simulink model "Leg"  (R2022a)
settings: Solver=VariableStepAuto  StartTime=0.0  StopTime=StopTime  FixedStep=0.001  MinStep=0.005  RelTol=1e-3
values from neighbouring files (symbols this model uses):
  l1 = 0.24    [thet_B.m]    (also in thet_S.m)
  l2 = 1.5    [thet_B.m]    (also in thet_S.m)
  l3 = 1.2    [thet_B.m]    (also in thet_S.m)
  l4 = 0.56    [thet_B.m]    (also in thet_S.m)
  s = size(theta_shag,1)    [Thetas.m]    (also in thet_B.m = size(sim_B.footPos,2); thet_P.m = size(sim_P.footPos,2); thet_S.m = size(simStates.footPos,2))
undefined symbols (not defined in the file or in its folder): L1, L2, L3, L4, m1, m2, m3, m4, mass_1, mass_2, mass_3, mass_4, X, Y, Z
libraries: nesl_utility x17, sm_lib x16
settings Model: Creator=boris_1863  LastModifiedBy=180
settings SolverCC: AlgebraicLoopSolver=TrustRegion
settings DataIOCC: MaxDataPoints=10000  ReturnWorkspaceOutputs=off  OutputTimes=0:0.01:StopTime
settings DebuggingCC: UnconnectedInputMsg=warning  UnconnectedOutputMsg=warning  UnconnectedLineMsg=warning  SFMachineParentedDataDiag=warning
settings RTWCC: DLArmComputeVersion=19.05
settings DiagnosticsConfigSet: SimMechanicsInvalidVisualProperty=none  SimMechanicsCrossSectionNullEdge=none  SimMechanicsUnconnectedFramePorts=none  SimMechanicsUnconnectedGeometryPorts=none  SimMechanicsRedundantBlock=none  SimMechanicsConflictingReferenceFrames=none  SimMechanicsRigidlyBoundBlock=none  SimMechanicsUnsatisfiedHighPriorityTargets=none  SimMechanicsJointTargetOverSpecification=none
settings ExplorerConfigSet: InternalSimMechanicsExplorerSettings="<ExplorerConfiguration><canonicalview>default</canonicalview><AnimationSetting><BasePlaybackSpeed>1.0</BasePlaybackSpeed><PlaybackSpeedFactor>4.0</PlaybackSpeedFactor></AnimationSetting><TilePanel><TileInfo><Tiles Columns=\"1\" Count=\"1\" Rows=\"1\"><Column Weight=\"1\"/><Row Weight=\"1\"/><Tile Height=\"1\" Width=\"1\" X=\"0\" Y=\"0\"/></Tiles></TileInfo><SceneInfo><SceneViewer><BGColor><R>1</R><G>1</G><B>1</B></BGColor><Camera><DoPerspective>off</DoPerspective><Position><X>0.0567000060216437882</X><Y>-1</Y><Z>0.046455009033208941</Z></Position><Center><X>0.0567000060216437882</X><Y>0</Y><Z>0.046455009033208941</Z></Center><Up><X>0</X><Y>-0</Y><Z>1</Z></Up><ViewLimDist>1</ViewLimDist><YLim>0.243616639058569923</YLim><XLim>0.23167689803025171</XLim></Camera></SceneViewer></SceneInfo></TilePanel><MechEditorPanel><Cameras/><GfxPanelCameraMap/><VideoCreator><PlaybackSpeedRatio>0.5</PlaybackSpeedRatio><FrameRate>60</FrameRate><VideoFormat>MPEG-4</VideoFormat><FrameSize>auto</FrameSize></VideoCreator></MechEditorPanel></ExplorerConfiguration>"

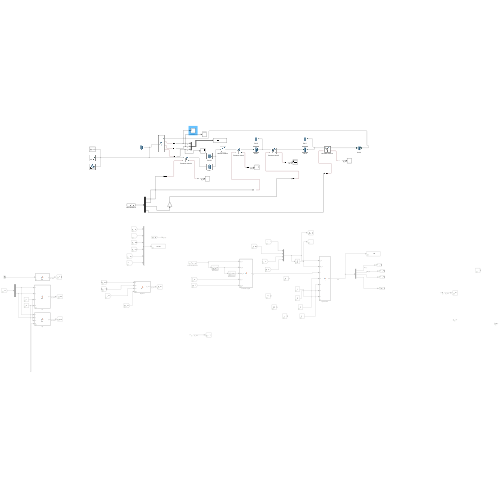
[thumbnail: Simulink's stored preview of the top-level diagram]
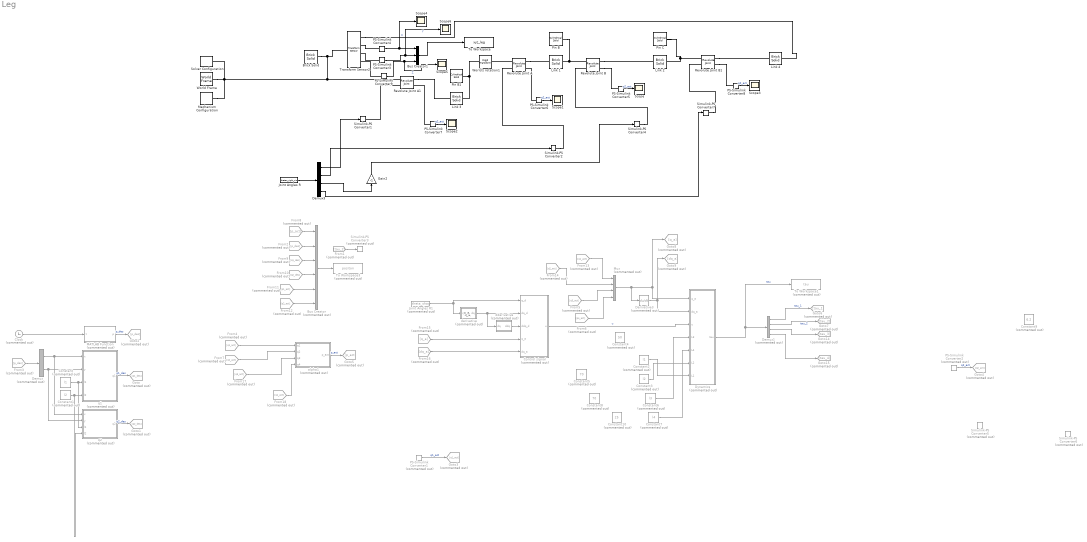
== system Leg ==
  note: q_a,
  note: q_a,
  Brick Solid : sm_lib/Body Elements/Brick Solid  GraphicAmbientColor=[0.15 0.15 0.15 1.0]  BasedOnType=Density  BrickDimensions=[0.12 0.12 0.12]  BrickDimensionUnits=m  CenterOfMass=[0 0 0]  CenterOfMassUnits=m  GraphicDiffuseColor=[0.2 0.2 0.2]  Density=1000  DensityUnits=kg/m^3  DoExposeReferenceFrame=on  GraphicEmissiveColor=[0.0 0.0 0.0 1.0]  ExportEntireGeometry=off  SerializedFrames=<Frames/>  MarkerShape=Sphere  MarkerSize=10  GraphicType=FromGeometry  InertiaType=CalculateFromGeometry  Mass=1  MassUnits=kg  MomentsOfInertia=[1 1 1]  MomentsOfInertiaUnits=kg*m^2  GraphicOpacity=1.0  ProductsOfInertia=[0 0 0]  ProductsOfInertiaUnits=kg*m^2  GraphicShininess=75  GraphicSpecularColor=[0.5 0.5 0.5 1.0]  GraphicVisPropType=SimpleVisualProperties
  Bus Creator : BusCreator  Commented=on  Inputs=6
  Bus Creator1 : BusCreator  Inputs=3
  Clock : Clock  Commented=on
  Constant : Constant  Commented=on  Value=l1
  Constant1 : Constant  Commented=on  Value=l2
  Constant10 : Constant  Commented=on  Value=25
  Constant2 : Constant  Commented=on  Value=l1
  Constant3 : Constant  Commented=on  Value=l2
  Constant4 : Constant  Commented=on  Value=50
  Constant5 : Constant  Commented=on  Value=70
  Constant6 : Constant  Commented=on  Value=l3
  Constant7 : Constant  Commented=on  Value=l4
  Constant8 : Constant  Commented=on  Value=70
  Constant9 : Constant  Commented=on  Value=6.2
  Control signal : MATLAB Function  Commented=on  TreatAsAtomicUnit=on
  Demux : Demux  Commented=on  Outputs=2
  Demux1 : Demux  Commented=on
  Demux3 : Demux
  Derivative3 : Derivative  Commented=on
  Dynamics : MATLAB Function  Commented=on  TreatAsAtomicUnit=on
  From1 : From  Commented=on  GotoTag=tau_2
  From10 : From  Commented=on  GotoTag=q2_des
  From11 : From  Commented=on  GotoTag=q1_act
  From12 : From  Commented=on  GotoTag=q2_act
  From13 : From  Commented=on  GotoTag=q1_act
  From14 : From  Commented=on  GotoTag=q2_act
  From15 : From  Commented=on  GotoTag=q_a
  From16 : From  Commented=on  GotoTag=dq_a
  From17 : From  Commented=on  GotoTag=q3_act
  From18 : From  Commented=on  GotoTag=q4_act
  From2 : From  Commented=on  GotoTag=p_des
  From3 : From  Commented=on  GotoTag=p_des
  From4 : From  Commented=on  GotoTag=q1_act
  From5 : From  Commented=on  GotoTag=q3_act
  From6 : From  Commented=on  GotoTag=q4_act
  From7 : From  Commented=on  GotoTag=q2_act
  From8 : From  Commented=on  GotoTag=p_act
  From9 : From  Commented=on  GotoTag=q1_des
  Gain2 : Gain  Gain=-1
  Goto : Goto  Commented=on  GotoTag=q1_des
  Goto1 : Goto  Commented=on  GotoTag=q2_des
  Goto14 : Goto  Commented=on  GotoTag=tau_3
  Goto15 : Goto  Commented=on  GotoTag=tau_4
  Goto2 : Goto  Commented=on  GotoTag=p_des
  Goto3 : Goto  Commented=on  GotoTag=q1_act
  Goto4 : Goto  Commented=on  GotoTag=q2_act
  Goto5 : Goto  Commented=on  GotoTag=p_act
  Goto6 : Goto  Commented=on  GotoTag=tau_1
  Goto7 : Goto  Commented=on  GotoTag=tau_2
  Goto8 : Goto  Commented=on  GotoTag=q_a
  Goto9 : Goto  Commented=on  GotoTag=dq_a
  Joint Angles R : FromWorkspace  VariableName=thetas_right_niz  OutputAfterFinalValue=Holding final value
  Joint Angles R1 : FromWorkspace  Commented=on  VariableName=theta_shag  OutputAfterFinalValue=Holding final value
  Link 1 : sm_lib/Body Elements/Brick Solid  GraphicAmbientColor=[0.15 0.15 0.15 1.0]  BasedOnType=Mass  BrickDimensions=BC  BrickDimensionUnits=m  CenterOfMass=[0 0 0]  CenterOfMassUnits=m  GraphicDiffuseColor=[0.6 0.6 1.0]  Density=1000  DensityUnits=kg/m^3  DoExposeReferenceFrame=off  GraphicEmissiveColor=[0.0 0.0 0.0 1.0]  ExportEntireGeometry=off  SerializedFrames=<Frames><Frame><Id>Frame1</Id><Value><Name>F1</Name><Origin><Source>GeometricFeature</Source><FeatureName>-x surface</FeatureName></Origin><PrimaryAxis><DefinedDirection>+Z</DefinedDirection><Source>ReferenceFrame</Source><SourceDirection>+Z</SourceDirection><FeatureName></FeatureName></PrimaryAxis><SecondaryAxis><DefinedDirection>+X</DefinedDirection><Source>ReferenceFrame</Source><SourceDirection>+X</SourceDirection><FeatureName></FeatureName></SecondaryAxis></Value></Frame><Frame><Id>Frame2</Id><Value><Name>F2</Name><Origin><Source>GeometricFeature</Source><FeatureName>+x surface</FeatureName></Origin><PrimaryAxis><DefinedDirection>+Z</DefinedDirection><Source>ReferenceFrame</Source><SourceDirection>+Z</SourceDirection><FeatureName></FeatureName></PrimaryAxis><SecondaryAxis><DefinedDirection>+X</DefinedDirection><Source>ReferenceFrame</Source><SourceDirection>+X</SourceDirection><FeatureName></FeatureName></SecondaryAxis></Value></Frame></Frames>  MarkerShape=Sphere  MarkerSize=10  GraphicType=FromGeometry  InertiaType=PointMass  Mass=mass_2  MassUnits=kg  MomentsOfInertia=[1 1 1]  MomentsOfInertiaUnits=kg*m^2  GraphicOpacity=1.0  ProductsOfInertia=[0 0 0]  ProductsOfInertiaUnits=kg*m^2  GraphicShininess=75  GraphicSpecularColor=[0.5 0.5 0.5 1.0]  GraphicVisPropType=SimpleVisualProperties
  Link 2 : sm_lib/Body Elements/Brick Solid  GraphicAmbientColor=[0.15 0.15 0.15 1.0]  BasedOnType=Mass  BrickDimensions=CD  BrickDimensionUnits=m  CenterOfMass=[0 0 0]  CenterOfMassUnits=m  GraphicDiffuseColor=[0.2 0.2 1.0]  Density=1000  DensityUnits=kg/m^3  DoExposeReferenceFrame=off  GraphicEmissiveColor=[0.0 0.0 0.0 1.0]  ExportEntireGeometry=off  SerializedFrames=<Frames><Frame><Id>Frame1</Id><Value><Name>F1</Name><Origin><Source>GeometricFeature</Source><FeatureName>-x surface</FeatureName></Origin><PrimaryAxis><DefinedDirection>+Z</DefinedDirection><Source>ReferenceFrame</Source><SourceDirection>+Z</SourceDirection><FeatureName></FeatureName></PrimaryAxis><SecondaryAxis><DefinedDirection>+X</DefinedDirection><Source>ReferenceFrame</Source><SourceDirection>+X</SourceDirection><FeatureName></FeatureName></SecondaryAxis></Value></Frame><Frame><Id>Frame2</Id><Value><Name>F2</Name><Origin><Source>GeometricFeature</Source><FeatureName>+x surface</FeatureName></Origin><PrimaryAxis><DefinedDirection>+Z</DefinedDirection><Source>ReferenceFrame</Source><SourceDirection>+Z</SourceDirection><FeatureName></FeatureName></PrimaryAxis><SecondaryAxis><DefinedDirection>+X</DefinedDirection><Source>ReferenceFrame</Source><SourceDirection>+X</SourceDirection><FeatureName></FeatureName></SecondaryAxis></Value></Frame></Frames>  MarkerShape=Sphere  MarkerSize=10  GraphicType=FromGeometry  InertiaType=PointMass  Mass=mass_3  MassUnits=kg  MomentsOfInertia=[1 1 1]  MomentsOfInertiaUnits=kg*m^2  GraphicOpacity=1.0  ProductsOfInertia=[0 0 0]  ProductsOfInertiaUnits=kg*m^2  GraphicShininess=75  GraphicSpecularColor=[0.5 0.5 0.5 1.0]  GraphicVisPropType=SimpleVisualProperties
  Link 3 : sm_lib/Body Elements/Brick Solid  GraphicAmbientColor=[0.15 0.15 0.15 1.0]  BasedOnType=Mass  BrickDimensions=AB  BrickDimensionUnits=m  CenterOfMass=[0 0 0]  CenterOfMassUnits=m  GraphicDiffuseColor=[0.6 0.6 1.0]  Density=1000  DensityUnits=kg/m^3  DoExposeReferenceFrame=off  GraphicEmissiveColor=[0.0 0.0 0.0 1.0]  ExportEntireGeometry=off  SerializedFrames=<Frames><Frame><Id>Frame1</Id><Value><Name>F1</Name><Origin><Source>GeometricFeature</Source><FeatureName>-x surface</FeatureName></Origin><PrimaryAxis><DefinedDirection>+Z</DefinedDirection><Source>ReferenceFrame</Source><SourceDirection>+Z</SourceDirection><FeatureName></FeatureName></PrimaryAxis><SecondaryAxis><DefinedDirection>+X</DefinedDirection><Source>ReferenceFrame</Source><SourceDirection>+X</SourceDirection><FeatureName></FeatureName></SecondaryAxis></Value></Frame><Frame><Id>Frame2</Id><Value><Name>F2</Name><Origin><Source>GeometricFeature</Source><FeatureName>+x surface</FeatureName></Origin><PrimaryAxis><DefinedDirection>+Z</DefinedDirection><Source>ReferenceFrame</Source><SourceDirection>+Z</SourceDirection><FeatureName></FeatureName></PrimaryAxis><SecondaryAxis><DefinedDirection>+X</DefinedDirection><Source>ReferenceFrame</Source><SourceDirection>+X</SourceDirection><FeatureName></FeatureName></SecondaryAxis></Value></Frame></Frames>  MarkerShape=Sphere  MarkerSize=10  GraphicType=FromGeometry  InertiaType=PointMass  Mass=mass_1  MassUnits=kg  MomentsOfInertia=[1 1 1]  MomentsOfInertiaUnits=kg*m^2  GraphicOpacity=1.0  ProductsOfInertia=[0 0 0]  ProductsOfInertiaUnits=kg*m^2  GraphicShininess=75  GraphicSpecularColor=[0.5 0.5 0.5 1.0]  GraphicVisPropType=SimpleVisualProperties
  Link 4 : sm_lib/Body Elements/Brick Solid  GraphicAmbientColor=[0.15 0.15 0.15 1.0]  BasedOnType=Mass  BrickDimensions=DE  BrickDimensionUnits=m  CenterOfMass=[0 0 0]  CenterOfMassUnits=m  GraphicDiffuseColor=[0.2 0.2 1.0]  Density=1000  DensityUnits=kg/m^3  DoExposeReferenceFrame=off  GraphicEmissiveColor=[0.0 0.0 0.0 1.0]  ExportEntireGeometry=off  SerializedFrames=<Frames><Frame><Id>Frame1</Id><Value><Name>F1</Name><Origin><Source>GeometricFeature</Source><FeatureName>-x surface</FeatureName></Origin><PrimaryAxis><DefinedDirection>+Z</DefinedDirection><Source>ReferenceFrame</Source><SourceDirection>+Z</SourceDirection><FeatureName></FeatureName></PrimaryAxis><SecondaryAxis><DefinedDirection>+X</DefinedDirection><Source>ReferenceFrame</Source><SourceDirection>+X</SourceDirection><FeatureName></FeatureName></SecondaryAxis></Value></Frame><Frame><Id>Frame2</Id><Value><Name>F2</Name><Origin><Source>GeometricFeature</Source><FeatureName>+x surface</FeatureName></Origin><PrimaryAxis><DefinedDirection>+Z</DefinedDirection><Source>ReferenceFrame</Source><SourceDirection>+Z</SourceDirection><FeatureName></FeatureName></PrimaryAxis><SecondaryAxis><DefinedDirection>+X</DefinedDirection><Source>ReferenceFrame</Source><SourceDirection>+X</SourceDirection><FeatureName></FeatureName></SecondaryAxis></Value></Frame></Frames>  MarkerShape=Sphere  MarkerSize=10  GraphicType=FromGeometry  InertiaType=PointMass  Mass=mass_4  MassUnits=kg  MomentsOfInertia=[1 1 1]  MomentsOfInertiaUnits=kg*m^2  GraphicOpacity=1.0  ProductsOfInertia=[0 0 0]  ProductsOfInertiaUnits=kg*m^2  GraphicShininess=75  GraphicSpecularColor=[0.5 0.5 0.5 1.0]  GraphicVisPropType=SimpleVisualProperties
  MATLAB Function : MATLAB Function  Commented=on  TreatAsAtomicUnit=on
  Mechanism Configuration : sm_lib/Utilities/Mechanism Configuration  UniformGravity=Constant  GravityVector=[0 0 -9.80665]  GravityUnits=m/s^2  LinearizationDelta=0.001  JointModeTransitionNonlinearIterations=2
  Mux : Mux  Commented=on
  PS-Simulink Converter1 : nesl_utility/PS-Simulink Converter  Commented=on  PhysicalDomain=network_engine_domain  SubClassName=ps_output  LeftPortType=input  RightPortType=output  PseudoPeriodic=off  Frequencies=[]  VectorFormat=1-D array  Unit=rad  AffineConversion=off
      settings: SourceProductBaseCode=SS,PW,VE
  PS-Simulink Converter2 : nesl_utility/PS-Simulink Converter  Commented=on  PhysicalDomain=network_engine_domain  SubClassName=ps_output  LeftPortType=input  RightPortType=output  PseudoPeriodic=off  Frequencies=[]  VectorFormat=1-D array  Unit=rad  AffineConversion=off
      settings: SourceProductBaseCode=SS,PW,VE
  PS-Simulink Converter3 : nesl_utility/PS-Simulink Converter  PhysicalDomain=network_engine_domain  SubClassName=ps_output  LeftPortType=input  RightPortType=output  PseudoPeriodic=off  Frequencies=[]  VectorFormat=1-D array  Unit=m  AffineConversion=off
      settings: SourceProductBaseCode=SS,PW,VE
  PS-Simulink Converter4 : nesl_utility/PS-Simulink Converter  PhysicalDomain=network_engine_domain  SubClassName=ps_output  LeftPortType=input  RightPortType=output  PseudoPeriodic=off  Frequencies=[]  VectorFormat=1-D array  Unit=m  AffineConversion=off
      settings: SourceProductBaseCode=SS,PW,VE
  PS-Simulink Converter{5..8} (4 alike) : nesl_utility/PS-Simulink Converter  PhysicalDomain=network_engine_domain  SubClassName=ps_output  LeftPortType=input  RightPortType=output  PseudoPeriodic=off  Frequencies=[]  VectorFormat=1-D array  Unit=rad  AffineConversion=off
      settings: SourceProductBaseCode=SS,PW,VE
  PS-Simulink Converter9 : nesl_utility/PS-Simulink Converter  PhysicalDomain=network_engine_domain  SubClassName=ps_output  LeftPortType=input  RightPortType=output  PseudoPeriodic=off  Frequencies=[]  VectorFormat=1-D array  Unit=m  AffineConversion=off
      settings: SourceProductBaseCode=SS,PW,VE
  Pin B : sm_lib/Body Elements/Cylindrical Solid  GraphicAmbientColor=[0.15 0.15 0.15 1.0]  BasedOnType=Density  CenterOfMass=[0 0 0]  CenterOfMassUnits=m  GraphicDiffuseColor=[0.6 0.6 1.0]  CylinderLength=0.11  CylinderLengthUnits=m  CylinderRadius=0.09/2  CylinderRadiusUnits=m  Density=0  DensityUnits=kg/m^3  DoExposeReferenceFrame=on  GraphicEmissiveColor=[0.0 0.0 0.0 1.0]  ExportEntireGeometry=off  SerializedFrames=<Frames/>  MarkerShape=Sphere  MarkerSize=10  GraphicType=FromGeometry  InertiaType=CalculateFromGeometry  Mass=1  MassUnits=kg  MomentsOfInertia=[1 1 1]  MomentsOfInertiaUnits=kg*m^2  GraphicOpacity=1.0  ProductsOfInertia=[0 0 0]  ProductsOfInertiaUnits=kg*m^2  GraphicShininess=75  GraphicSpecularColor=[0.5 0.5 0.5 1.0]  GraphicVisPropType=SimpleVisualProperties
  Pin B1 : sm_lib/Body Elements/Cylindrical Solid  GraphicAmbientColor=[0.15 0.15 0.15 1.0]  BasedOnType=Density  CenterOfMass=[0 0 0]  CenterOfMassUnits=m  GraphicDiffuseColor=[0.6 0.6 1.0]  CylinderLength=0.11  CylinderLengthUnits=m  CylinderRadius=0.09/2  CylinderRadiusUnits=m  Density=0  DensityUnits=kg/m^3  DoExposeReferenceFrame=on  GraphicEmissiveColor=[0.0 0.0 0.0 1.0]  ExportEntireGeometry=off  SerializedFrames=<Frames/>  MarkerShape=Sphere  MarkerSize=10  GraphicType=FromGeometry  InertiaType=CalculateFromGeometry  Mass=1  MassUnits=kg  MomentsOfInertia=[1 1 1]  MomentsOfInertiaUnits=kg*m^2  GraphicOpacity=1.0  ProductsOfInertia=[0 0 0]  ProductsOfInertiaUnits=kg*m^2  GraphicShininess=75  GraphicSpecularColor=[0.5 0.5 0.5 1.0]  GraphicVisPropType=SimpleVisualProperties
  Pin C : sm_lib/Body Elements/Cylindrical Solid  GraphicAmbientColor=[0.15 0.15 0.15 1.0]  BasedOnType=Density  CenterOfMass=[0 0 0]  CenterOfMassUnits=m  GraphicDiffuseColor=[0.2 0.2 1.0]  CylinderLength=0.1  CylinderLengthUnits=m  CylinderRadius=0.08/2  CylinderRadiusUnits=m  Density=0  DensityUnits=kg/m^3  DoExposeReferenceFrame=on  GraphicEmissiveColor=[0.0 0.0 0.0 1.0]  ExportEntireGeometry=off  SerializedFrames=<Frames/>  MarkerShape=Sphere  MarkerSize=10  GraphicType=FromGeometry  InertiaType=CalculateFromGeometry  Mass=1  MassUnits=kg  MomentsOfInertia=[1 1 1]  MomentsOfInertiaUnits=kg*m^2  GraphicOpacity=1.0  ProductsOfInertia=[0 0 0]  ProductsOfInertiaUnits=kg*m^2  GraphicShininess=75  GraphicSpecularColor=[0.5 0.5 0.5 1.0]  GraphicVisPropType=SimpleVisualProperties
  Revolute Joint A : sm_lib/Joints/Revolute Joint  JointMode=Normal  SenseConstraintForce=off  SenseConstraintForceX=off  SenseConstraintForceY=off  SenseConstraintForceZ=off  SenseConstraintTorque=off  SenseConstraintTorqueX=off  SenseConstraintTorqueY=off  SenseConstraintTorqueZ=off  SenseTotalForce=off  SenseTotalForceX=off  SenseTotalForceY=off  SenseTotalForceZ=off  SenseTotalTorque=off  SenseTotalTorqueX=off  SenseTotalTorqueY=off  SenseTotalTorqueZ=off  CompositeWrenchDir=FollowerOnBase  CompositeWrenchFrame=BaseFrame  EquilibriumPosition=0  EquilibriumPositionUnits=deg  SpringStiffness=0  SpringStiffnessUnits=N*m/deg  DampingCoefficient=0  DampingCoefficientUnits=N*m/(rad/s)  TorqueActuationMode=ComputedTorque  MotionActuationMode=InputMotion  SensePosition=on  SenseVelocity=off  SenseAcceleration=off  SenseTorqueForce=off  SenseLowerLimitTorqueForce=off  SenseUpperLimitTorqueForce=off  LowerLimitSpecify=off  LowerLimitBound=0  LowerLimitBoundUnits=deg  LowerLimitStiffness=1e4  LowerLimitStiffnessUnits=N*m/deg  LowerLimitDamping=10  LowerLimitDampingUnits=N*m/(deg/s)  LowerLimitTransitionRegionWidth=0.1  LowerLimitTransitionRegionWidthUnits=deg  UpperLimitSpecify=off  UpperLimitBound=90  UpperLimitBoundUnits=deg  UpperLimitStiffness=1e4  UpperLimitStiffnessUnits=N*m/deg  UpperLimitDamping=10  UpperLimitDampingUnits=N*m/(deg/s)  UpperLimitTransitionRegionWidth=0.1  UpperLimitTransitionRegionWidthUnits=deg  PositionTargetSpecify=off  PositionTargetPriority=High  PositionTargetValue=-2.6  PositionTargetValueUnits=rad  VelocityTargetSpecify=off  VelocityTargetPriority=High  VelocityTargetValue=0  VelocityTargetValueUnits=deg/s
  Revolute Joint A1 : sm_lib/Joints/Revolute Joint  JointMode=Normal  SenseConstraintForce=off  SenseConstraintForceX=off  SenseConstraintForceY=off  SenseConstraintForceZ=off  SenseConstraintTorque=off  SenseConstraintTorqueX=off  SenseConstraintTorqueY=off  SenseConstraintTorqueZ=off  SenseTotalForce=off  SenseTotalForceX=off  SenseTotalForceY=off  SenseTotalForceZ=off  SenseTotalTorque=off  SenseTotalTorqueX=off  SenseTotalTorqueY=off  SenseTotalTorqueZ=off  CompositeWrenchDir=FollowerOnBase  CompositeWrenchFrame=BaseFrame  EquilibriumPosition=0  EquilibriumPositionUnits=deg  SpringStiffness=0  SpringStiffnessUnits=N*m/deg  DampingCoefficient=0  DampingCoefficientUnits=N*m/(rad/s)  TorqueActuationMode=ComputedTorque  MotionActuationMode=InputMotion  SensePosition=on  SenseVelocity=off  SenseAcceleration=off  SenseTorqueForce=off  SenseLowerLimitTorqueForce=off  SenseUpperLimitTorqueForce=off  LowerLimitSpecify=off  LowerLimitBound=0  LowerLimitBoundUnits=deg  LowerLimitStiffness=1e4  LowerLimitStiffnessUnits=N*m/deg  LowerLimitDamping=10  LowerLimitDampingUnits=N*m/(deg/s)  LowerLimitTransitionRegionWidth=0.1  LowerLimitTransitionRegionWidthUnits=deg  UpperLimitSpecify=off  UpperLimitBound=90  UpperLimitBoundUnits=deg  UpperLimitStiffness=1e4  UpperLimitStiffnessUnits=N*m/deg  UpperLimitDamping=10  UpperLimitDampingUnits=N*m/(deg/s)  UpperLimitTransitionRegionWidth=0.1  UpperLimitTransitionRegionWidthUnits=deg  PositionTargetSpecify=off  PositionTargetPriority=High  PositionTargetValue=-2.6  PositionTargetValueUnits=rad  VelocityTargetSpecify=off  VelocityTargetPriority=High  VelocityTargetValue=0  VelocityTargetValueUnits=deg/s
  Revolute Joint B : sm_lib/Joints/Revolute Joint  JointMode=Normal  SenseConstraintForce=off  SenseConstraintForceX=off  SenseConstraintForceY=off  SenseConstraintForceZ=off  SenseConstraintTorque=off  SenseConstraintTorqueX=off  SenseConstraintTorqueY=off  SenseConstraintTorqueZ=off  SenseTotalForce=off  SenseTotalForceX=off  SenseTotalForceY=off  SenseTotalForceZ=off  SenseTotalTorque=off  SenseTotalTorqueX=off  SenseTotalTorqueY=off  SenseTotalTorqueZ=off  CompositeWrenchDir=FollowerOnBase  CompositeWrenchFrame=BaseFrame  EquilibriumPosition=0  EquilibriumPositionUnits=deg  SpringStiffness=0  SpringStiffnessUnits=N*m/deg  DampingCoefficient=0  DampingCoefficientUnits=N*m/(rad/s)  TorqueActuationMode=ComputedTorque  MotionActuationMode=InputMotion  SensePosition=on  SenseVelocity=off  SenseAcceleration=off  SenseTorqueForce=off  SenseLowerLimitTorqueForce=off  SenseUpperLimitTorqueForce=off  LowerLimitSpecify=off  LowerLimitBound=0  LowerLimitBoundUnits=deg  LowerLimitStiffness=1e4  LowerLimitStiffnessUnits=N*m/deg  LowerLimitDamping=10  LowerLimitDampingUnits=N*m/(deg/s)  LowerLimitTransitionRegionWidth=0.1  LowerLimitTransitionRegionWidthUnits=deg  UpperLimitSpecify=off  UpperLimitBound=90  UpperLimitBoundUnits=deg  UpperLimitStiffness=1e4  UpperLimitStiffnessUnits=N*m/deg  UpperLimitDamping=10  UpperLimitDampingUnits=N*m/(deg/s)  UpperLimitTransitionRegionWidth=0.1  UpperLimitTransitionRegionWidthUnits=deg  PositionTargetSpecify=off  PositionTargetPriority=High  PositionTargetValue=1.81  PositionTargetValueUnits=rad  VelocityTargetSpecify=off  VelocityTargetPriority=High  VelocityTargetValue=0  VelocityTargetValueUnits=deg/s
  Revolute Joint B1 : sm_lib/Joints/Revolute Joint  JointMode=Normal  SenseConstraintForce=off  SenseConstraintForceX=off  SenseConstraintForceY=off  SenseConstraintForceZ=off  SenseConstraintTorque=off  SenseConstraintTorqueX=off  SenseConstraintTorqueY=off  SenseConstraintTorqueZ=off  SenseTotalForce=off  SenseTotalForceX=off  SenseTotalForceY=off  SenseTotalForceZ=off  SenseTotalTorque=off  SenseTotalTorqueX=off  SenseTotalTorqueY=off  SenseTotalTorqueZ=off  CompositeWrenchDir=FollowerOnBase  CompositeWrenchFrame=BaseFrame  EquilibriumPosition=0  EquilibriumPositionUnits=deg  SpringStiffness=0  SpringStiffnessUnits=N*m/deg  DampingCoefficient=0  DampingCoefficientUnits=N*m/(rad/s)  TorqueActuationMode=ComputedTorque  MotionActuationMode=InputMotion  SensePosition=on  SenseVelocity=off  SenseAcceleration=off  SenseTorqueForce=off  SenseLowerLimitTorqueForce=off  SenseUpperLimitTorqueForce=off  LowerLimitSpecify=off  LowerLimitBound=175  LowerLimitBoundUnits=deg  LowerLimitStiffness=1e4  LowerLimitStiffnessUnits=N*m/deg  LowerLimitDamping=10  LowerLimitDampingUnits=N*m/(deg/s)  LowerLimitTransitionRegionWidth=0.1  LowerLimitTransitionRegionWidthUnits=deg  UpperLimitSpecify=off  UpperLimitBound=175  UpperLimitBoundUnits=deg  UpperLimitStiffness=1e4  UpperLimitStiffnessUnits=N*m/deg  UpperLimitDamping=10  UpperLimitDampingUnits=N*m/(deg/s)  UpperLimitTransitionRegionWidth=0.1  UpperLimitTransitionRegionWidthUnits=deg  PositionTargetSpecify=off  PositionTargetPriority=High  PositionTargetValue=1.81  PositionTargetValueUnits=rad  VelocityTargetSpecify=off  VelocityTargetPriority=High  VelocityTargetValue=0  VelocityTargetValueUnits=deg/s
  Scope{,1..6} (7 alike) : Scope
  Simulink-PS Converter{1..2,4,7} (4 alike) : nesl_utility/Simulink-PS Converter  PhysicalDomain=network_engine_domain  SubClassName=ps_input  LeftPortType=input  RightPortType=output  PseudoPeriodic=off  Frequencies=[]  NoiseDistribution=none  NoiseParameters=[]  Unit=rad  AffineConversion=off  FilteringAndDerivatives=filter  SimscapeFilterOrder=2  InputFilterTimeConstant=0.005  UdotUserProvided=0
      settings: SourceProductBaseCode=SS,PW,VE
  Simulink-PS Converter3 : nesl_utility/Simulink-PS Converter  Commented=on  PhysicalDomain=network_engine_domain  SubClassName=ps_input  LeftPortType=input  RightPortType=output  PseudoPeriodic=off  Frequencies=[]  NoiseDistribution=none  NoiseParameters=[]  Unit=N*m  AffineConversion=off  FilteringAndDerivatives=provide  SimscapeFilterOrder=2  InputFilterTimeConstant=0.001  UdotUserProvided=0
      settings: SourceProductBaseCode=SS,PW,VE
  Simulink-PS Converter5 : nesl_utility/Simulink-PS Converter  Commented=on  PhysicalDomain=network_engine_domain  SubClassName=ps_input  LeftPortType=input  RightPortType=output  PseudoPeriodic=off  Frequencies=[]  NoiseDistribution=none  NoiseParameters=[]  Unit=rad  AffineConversion=off  FilteringAndDerivatives=filter  SimscapeFilterOrder=2  InputFilterTimeConstant=0.005  UdotUserProvided=0
      settings: SourceProductBaseCode=SS,PW,VE
  Simulink-PS Converter6 : nesl_utility/Simulink-PS Converter  Commented=on  PhysicalDomain=network_engine_domain  SubClassName=ps_input  LeftPortType=input  RightPortType=output  PseudoPeriodic=off  Frequencies=[]  NoiseDistribution=none  NoiseParameters=[]  Unit=rad  AffineConversion=off  FilteringAndDerivatives=filter  SimscapeFilterOrder=2  InputFilterTimeConstant=0.005  UdotUserProvided=0
      settings: SourceProductBaseCode=SS,PW,VE
  Solver Configuration : nesl_utility/Solver Configuration  PhysicalDomain=network_engine_domain  SubClassName=solver  LeftPortType=input  RightPortType=generic  Tones=[]  Harmonics=[]  SimulateNoise=off  Profile=off  UseLocalSampling=off  EnableSwitchedLinearOptims=on  FrequencyDomain=off  UseCCode=off  RelTol=0.001  AbsTol=1e-06  MinStep=1e-09  ToWorkspace=off  RevertToSquareIcSolve=off  NumHomotopyIterations=100  PhasorMode=off  PhasorModeNumHarmonics=1  IndexReductionMethod=DerivativeReplacement  DoDC=off  ResidualTolerance=1e-09  UseLocalSolver=off  LocalSolverChoice=NE_BACKWARD_EULER_ADVANCER  LocalSolverSampleTime=0.001  DoFixedCost=off  MaxNonlinIter=3  MaxModeIter=2  ComputeImpulses=off  ImpulseIterations=2  LinearAlgebra=Sparse  LinearAlgebraNumThread=0  EquationFormulation=NE_TIME_EF  DelaysMemoryBudget=1024  AutomaticFiltering=on  FilteringTimeConstant=0.001  PartitionStorageMethod=AS_NEEDED  PartitionMemoryBudget=1024  PartitionMethod=FAST
      settings: SourceProductBaseCode=SS,PW,VE
  To Workspace : ToWorkspace  VariableName=xyz_leg  SaveFormat=Timeseries  SampleTime=-1
  To Workspace1 : ToWorkspace  Commented=on  VariableName=tau  SaveFormat=Timeseries  SampleTime=-1
  To Workspace3 : ToWorkspace  Commented=on  VariableName=positon  SaveFormat=Timeseries  SampleTime=-1
  Transform Sensor2 : sm_lib/Frames and Transforms/Transform Sensor  MeasurementFrame=World  SenseAngle=off  SenseAxis=off  SenseAngle1=off  SenseAngle2=off  SenseAngle3=off  SenseQ=off  SenseR=off  SenseOmegaX=off  SenseOmegaY=off  SenseOmegaZ=off  SenseOmega1=off  SenseOmega2=off  SenseOmega3=off  SenseQDot=off  SenseRDot=off  SenseAlphaX=off  SenseAlphaY=off  SenseAlphaZ=off  SenseAlpha1=off  SenseAlpha2=off  SenseAlpha3=off  SenseQDDot=off  SenseRDDot=off  SenseX=on  SenseY=on  SenseZ=on  SenseRad=off  SenseAzim=off  SenseDist=off  SenseInc=off  SenseXDot=off  SenseYDot=off  SenseZDot=off  SenseRadDot=off  SenseAzimDot=off  SenseDistDot=off  SenseIncDot=off  SenseXDDot=off  SenseYDDot=off  SenseZDDot=off  SenseRadDDot=off  SenseAzimDDot=off  SenseDistDDot=off  SenseIncDDot=off
  World Frame : sm_lib/Frames and Transforms/World Frame
  World's rotation1 : sm_lib/Frames and Transforms/Rigid Transform  TranslationMethod=None  TranslationStandardOffset=0  TranslationLengthUnit=m  TranslationStandardAxis=+Z  TranslationCartesianOffset=[0 0 0]  TranslationROffset=0  TranslationROffsetUnits=m  TranslationZOffset=0  TranslationZOffsetUnits=m  TranslationThetaOffset=0  TranslationThetaOffsetUnits=deg  RotationMethod=StandardAxis  RotationAngleUnits=deg  RotationStandardAxis=+X  RotationAngle=90  RotationArbitraryAxis=[0 0 1]  FollAlignAxisA=+X  BaseAlignAxisA=+Y  FollAlignAxisB=+Y  BaseAlignAxisB=+Z  RotationSequenceAxes=FollowerAxes  RotationSequence=XYX  RotationSequenceAngles=[0 0 0]  RotationSequenceAnglesUnits=deg  RotationMatrix=[1 0 0; 0 1 0; 0 0 1]
  alpha1 : MATLAB Function  Commented=on  TreatAsAtomicUnit=on
  dderivative : Subsystem  Commented=on
  derivative : Subsystem  Commented=on
  q1 : MATLAB Function  Commented=on  TreatAsAtomicUnit=on
  q2 : MATLAB Function  Commented=on  TreatAsAtomicUnit=on
  wires:
  Demux3/1 -> Simulink-PS Converter1/1
  q2/1(q2) -> Goto1/1  "q2_des"
  PS-Simulink Converter1/1 -> Goto3/1  "q1_act"
  Demux/1 -> q2/1(x), q1/1(x)
  Clock/1 -> MATLAB Function/1(t)
  MATLAB Function/1(p) -> Goto2/1  "p_des"
  From1/1 -> Simulink-PS Converter3/1
  q1/1(q1) -> Goto/1  "q1_des"
  Bus Creator/1 -> To Workspace3/1
  Demux/2 -> q2/2(y), q1/2(y)
  Constant/1 -> q2/3(l1), q1/3(l1)
  Constant1/1 -> q2/4(l2), q1/4(l2)
  From3/1 -> Demux/1
  PS-Simulink Converter2/1 -> Goto4/1  "q2_act"
  From4/1 -> alpha1/1(q1)
  From7/1 -> alpha1/2(q2)
  alpha1/1(p_act) -> Goto5/1  "p_act"
  From8/1 -> Bus Creator/1
  From2/1 -> Bus Creator/2
  From9/1 -> Bus Creator/3
  From10/1 -> Bus Creator/4
  From11/1 -> Bus Creator/5
  From12/1 -> Bus Creator/6
  From13/1 -> Mux/1
  Dynamics/1(tau) -> To Workspace1/1, Demux1/1  "tau"
  Demux1/1 -> Goto6/1  "tau_1"
  Demux1/2 -> Goto7/1  "tau_2"
  From14/1 -> Mux/2
  Mux/1 -> Dynamics/1(q_a), Goto8/1, Derivative3/1
  Derivative3/1 -> Goto9/1, Dynamics/2(dq_a)
  Joint Angles R1/1 -> derivative/1(q), Control signal/1(q_d)
  derivative/1(dq) -> Control signal/2(dq_d), dderivative/1(dq)
  From15/1 -> Control signal/4(q_a)
  From16/1 -> Control signal/5(dq_a)
  Control signal/1(u) -> Dynamics/3(u)  "u"
  dderivative/1(ddq) -> Control signal/3(ddq_d)
  PS-Simulink Converter5/1 -> Scope/1  "q2_act"
  PS-Simulink Converter6/1 -> Scope1/1  "q2_act"
  PS-Simulink Converter7/1 -> Scope2/1  "q2_act"
  PS-Simulink Converter8/1 -> Scope3/1  "q2_act"
  Joint Angles R/1 -> Demux3/1
  Demux3/3 -> Gain2/1
  From17/1 -> alpha1/3(q3)
  From18/1 -> alpha1/4(q4)
  From5/1 -> Mux/3
  From6/1 -> Mux/4
  Constant6/1 -> Dynamics/4(L3)
  Demux1/3 -> Goto14/1
  Demux1/4 -> Goto15/1
  Demux3/2 -> Simulink-PS Converter2/1
  Gain2/1 -> Simulink-PS Converter4/1
  Demux3/4 -> Simulink-PS Converter7/1
  Constant2/1 -> Dynamics/7(L1)
  Constant3/1 -> Dynamics/6(L2)
  Constant7/1 -> Dynamics/5(L4)
  Bus Creator1/1 -> To Workspace/1
  PS-Simulink Converter3/1 -> Scope6/1, Bus Creator1/2  "Y"
  PS-Simulink Converter9/1 -> Scope5/1, Bus Creator1/3  "Z"
  PS-Simulink Converter4/1 -> Scope4/1, Bus Creator1/1  "X"
  connections:
  Brick Solid/RConn1 -- Transform Sensor2/LConn1 -- World Frame/RConn1 -- Solver Configuration/RConn1 -- Mechanism Configuration/RConn1 -- Revolute Joint A1/LConn1
  Pin C/RConn1 -- Revolute Joint B1/LConn1 -- Link 2/RConn1
  Revolute Joint A/RConn1 -- Link 1/LConn1
  Revolute Joint B/RConn1 -- Link 2/LConn1
  Revolute Joint B/LConn1 -- Pin B/RConn1 -- Link 1/RConn1
  PS-Simulink Converter3/LConn1 -- Transform Sensor2/RConn3
  Transform Sensor2/RConn2 -- PS-Simulink Converter4/LConn1
  Revolute Joint A/LConn1 -- World's rotation1/RConn1
  Revolute Joint A1/RConn1 -- Link 3/LConn1
  Revolute Joint B/RConn2 -- PS-Simulink Converter5/LConn1
  PS-Simulink Converter6/LConn1 -- Revolute Joint A/RConn2
  PS-Simulink Converter7/LConn1 -- Revolute Joint A1/RConn2
  Revolute Joint A1/LConn2 -- Simulink-PS Converter1/RConn1
  World's rotation1/LConn1 -- Link 3/RConn1 -- Pin B1/RConn1
  Transform Sensor2/RConn1 -- Link 4/RConn1
  Revolute Joint B1/RConn2 -- PS-Simulink Converter8/LConn1
  Revolute Joint B1/RConn1 -- Link 4/LConn1
  Simulink-PS Converter2/RConn1 -- Revolute Joint A/LConn2
  Simulink-PS Converter4/RConn1 -- Revolute Joint B/LConn2
  Simulink-PS Converter7/RConn1 -- Revolute Joint B1/LConn2
  PS-Simulink Converter9/LConn1 -- Transform Sensor2/RConn4

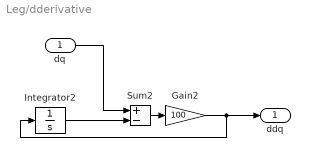
== system Leg/dderivative ==
  dq : Inport
  Gain2 : Gain  Gain=100
  Integrator2 : Integrator
  Sum2 : Sum  Inputs=+-
  ddq : Outport
  wires:
  dq/1 -> Sum2/1
  Integrator2/1 -> Sum2/2
  Sum2/1 -> Gain2/1
  Gain2/1 -> ddq/1, Integrator2/1

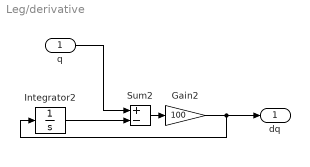
== system Leg/derivative ==
  q : Inport
  Gain2 : Gain  Gain=100
  Integrator2 : Integrator
  Sum2 : Sum  Inputs=+-
  dq : Outport
  wires:
  q/1 -> Sum2/1
  Integrator2/1 -> Sum2/2
  Sum2/1 -> Gain2/1
  Gain2/1 -> dq/1, Integrator2/1

== matlab function Leg/q2 ==
  data: x input; q2 output; y input; l1 input; l2 input
function q2 = fcn(x,y,l1,l2)
argument=(l1^2+l2^2-x^2-y^2)/(2*l1*l2);
beta = acos(argument);
q2 = -pi + beta;

== matlab function Leg/MATLAB Function ==
  data: t input; p output
function p = fcn(t)
p = [0.4*sin(1*t)+1.6;...
     0.2*cos(1*t)-0.7];

== matlab function Leg/q1 ==
  data: x input; q1 output; y input; l1 input; l2 input
function q1 = fcn(x,y,l1,l2)
argument = (x^2+y^2+l1^2-l2^2)/(2*l1*sqrt(x^2+y^2));
alpha = acos(argument);
gamma = atan2(y,x);
q1 = gamma + alpha;

== matlab function Leg/alpha1 ==
  data: q1 input; p_act output; q2 input; q3 input; q4 input; L1 parameter; L2 parameter; L3 parameter; L4 parameter
function p_act = fcn(q1,q2,q3,q4,L1, L2, L3, L4)
p_act = my_pr(q1,q2,q3,q4,L1,L2,L3,L4);

== matlab function Leg/Dynamics ==
  data: q_a input; dq_a input; u input; m3 parameter; L3 input; tau output; L4 input; m2 parameter; m1 parameter; L2 input; L1 input; m4 parameter
function tau = fcn(q_a,dq_a,u,m3,L3,L4, m2, m1, L2, L1, m4)
q10 = [1 0 0 0]*q_a;
q20 = [0 1 0 0]*q_a;
q30 = [0 0 1 0]*q_a;
q40 = [0 0 0 1]*q_a;

w1 = [1 0 0 0]*dq_a;
w2 = [0 1 0 0]*dq_a;
w3 = [0 0 1 0]*dq_a;
w4 = [0 0 0 1]*dq_a;

% g=9.80665;%gravitation
% 
% M=[0.25*m1*l1^2+m2*(l1^2+l1*l2*cos(q2)+0.25*l2^2) m2*(0.5*l1*l2*cos(q2)+0.25*l2^2);...
%     m2*(0.5*l1*l2*cos(q2)+0.25*l2^2) 0.25*m2*l2^2];
% C=[-0.5*m2*l1*l2*sin(q2)*(2*w1*w2+w2^2);...
%     0.5*m2*l1*l2*sin(q2)*w1^2];
% N=[(0.5*m1+m2)*g*l1*cos(q1)+0.5*m2*g*l2*cos(q1+q2);...
%     0.5*m2*g*l2*cos(q1+q2)];



 
M =[(L1^2*m1)/4 + L1^2*m2 + L1^2*m3 + (L2^2*m2)/8 + L1^2*m4 + (L2^2*m3)/2 + (L2^2*m4)/2 + (L3^2*m3)/8 + (L3^2*m4)/2 + (L4^2*m4)/8 + (L2^2*m2*cos(2*q20))/8 + (L2^2*m3*cos(2*q20))/2 + (L2^2*m4*cos(2*q20))/2 + (L4^2*m4*cos(2*q20 + 2*q30 + 2*q40))/8 + (L3^2*m3*cos(2*q20 + 2*q30))/8 + (L3^2*m4*cos(2*q20 + 2*q30))/2 + L1*L3*m3*cos(q20 + q30) + 2*L1*L3*m4*cos(q20 + q30) + (L2*L4*m4*cos(q30 + q40))/2 + L1*L2*m2*cos(q20) + 2*L1*L2*m3*cos(q20) + 2*L1*L2*m4*cos(q20) + (L2*L3*m3*cos(q30))/2 + L2*L3*m4*cos(q30) + (L3*L4*m4*cos(q40))/2 + (L3*L4*m4*cos(2*q20 + 2*q30 + q40))/2 + (L2*L3*m3*cos(2*q20 + q30))/2 + L2*L3*m4*cos(2*q20 + q30) + L1*L4*m4*cos(q20 + q30 + q40) + (L2*L4*m4*cos(2*q20 + q30 + q40))/2 0 0 0;...
    0 (L2^2*m2)/8 + (L2^2*m3)/2 + (L2^2*m4)/2 + (L3^2*m3)/8 + (L3^2*m4)/2 + (L4^2*m4)/8 - (L2^2*m2*cos(2*q20))/8 - (L2^2*m3*cos(2*q20))/2 - (L2^2*m4*cos(2*q20))/2 - (L4^2*m4*cos(2*q20 + 2*q30 + 2*q40))/8 - (L3^2*m3*cos(2*q20 + 2*q30))/8 - (L3^2*m4*cos(2*q20 + 2*q30))/2 + (L2*L4*m4*cos(q30 + q40))/2 + (L2*L3*m3*cos(q30))/2 + L2*L3*m4*cos(q30) + (L3*L4*m4*cos(q40))/2 - (L3*L4*m4*cos(2*q20 + 2*q30 + q40))/2 - (L2*L3*m3*cos(2*q20 + q30))/2 - L2*L3*m4*cos(2*q20 + q30) - (L2*L4*m4*cos(2*q20 + q30 + q40))/2 (L3^2*m3)/8 + (L3^2*m4)/2 + (L4^2*m4)/8 - (L4^2*m4*cos(2*q20 + 2*q30 + 2*q40))/8 - (L3^2*m3*cos(2*q20 + 2*q30))/8 - (L3^2*m4*cos(2*q20 + 2*q30))/2 + (L2*L4*m4*cos(q30 + q40))/4 + (L2*L3*m3*cos(q30))/4 + (L2*L3*m4*cos(q30))/2 + (L3*L4*m4*cos(q40))/2 - (L3*L4*m4*cos(2*q20 + 2*q30 + q40))/2 - (L2*L3*m3*cos(2*q20 + q30))/4 - (L2*L3*m4*cos(2*q20 + q30))/2 - (L2*L4*m4*cos(2*q20 + q30 + q40))/4 (L4*m4*(L4 - 2*L2*cos(2*q20 + q30 + q40) + 2*L2*cos(q30 + q40) + 2*L3*cos(q40) - 2*L3*cos(2*q20 + 2*q30 + q40) - L4*cos(2*q20 + 2*q30 + 2*q40)))/8;...
    0 (L3^2*m3)/8 + (L3^2*m4)/2 + (L4^2*m4)/8 - (L4^2*m4*cos(2*q20 + 2*q30 + 2*q40))/8 - (L3^2*m3*cos(2*q20 + 2*q30))/8 - (L3^2*m4*cos(2*q20 + 2*q30))/2 + (L2*L4*m4*cos(q30 + q40))/4 + (L2*L3*m3*cos(q30))/4 + (L2*L3*m4*cos(q30))/2 + (L3*L4*m4*cos(q40))/2 - (L3*L4*m4*cos(2*q20 + 2*q30 + q40))/2 - (L2*L3*m3*cos(2*q20 + q30))/4 - (L2*L3*m4*cos(2*q20 + q30))/2 - (L2*L4*m4*cos(2*q20 + q30 + q40))/4 (L3^2*m3)/8 + (L3^2*m4)/2 + (L4^2*m4)/8 - (L4^2*m4*cos(2*q20 + 2*q30 + 2*q40))/8 - (L3^2*m3*cos(2*q20 + 2*q30))/8 - (L3^2*m4*cos(2*q20 + 2*q30))/2 + (L3*L4*m4*cos(q40))/2 - (L3*L4*m4*cos(2*q20 + 2*q30 + q40))/2 (L4*m4*(L4 + 2*L3*cos(q40) - 2*L3*cos(2*q20 + 2*q30 + q40) - L4*cos(2*q20 + 2*q30 + 2*q40)))/8;...
    0 (L4*m4*(L4 - 2*L2*cos(2*q20 + q30 + q40) + 2*L2*cos(q30 + q40) + 2*L3*cos(q40) - 2*L3*cos(2*q20 + 2*q30 + q40) - L4*cos(2*q20 + 2*q30 + 2*q40)))/8 (L4*m4*(L4 + 2*L3*cos(q40) - 2*L3*cos(2*q20 + 2*q30 + q40) - L4*cos(2*q20 + 2*q30 + 2*q40)))/8 -(L4^2*m4*(cos(2*q20 + 2*q30 + 2*q40) - 1))/8];
 
 
N =[0;...
    g*((L4*m4*cos(q20 + q30 + q40))/2 + (L2*m3*cos(q20 + q30))/2 + L3*m4*cos(q20 + q30) + (L2*m2*cos(q20))/2 + L2*m3*cos(q20) + L2*m4*cos(q20));...
    g*((L4*m4*cos(q20 + q30 + q40))/2 + (L2*m3*cos(q20 + q30))/2 + L3*m4*cos(q20 + q30));...
    (L4*g*m4*cos(q20 + q30 + q40))/2];
 


% M=M0;
% M = subs(M,m1,m01);
% M = subs(M,m2,m02);
% M = subs(M,m3,m03);
% M = subs(M,m4,m04);
% 
% M = subs(M,L1,l1);
% M = subs(M,L2,l2);
% M = subs(M,L3,l3);
% M = subs(M,L4,l4);
% 
% M = subs(M,q1,q10);
% M = subs(M,q2,q20);
% M = subs(M,q3,q30);
% M = subs(M,q4,q40);


% N = subs(N,m1,m01);
% N = subs(N,m2,m02);
% N = subs(N,m3,m03);
% N = subs(N,m4,m04);
% 
% N = subs(N,L1,l1);
% N = subs(N,L2,l2);
% N = subs(N,L3,l3);
% N = subs(N,L4,l4);
% 
% N = subs(N,q1,q10);
% N = subs(N,q2,q20);
% N = subs(N,q3,q30);
% N = subs(N,q4,q40);


% C = subs(C,m1,m01);
% C = subs(C,m2,m02);
% C = subs(C,m3,m03);
% C = subs(C,m4,m04);
% 
% C = subs(C,L1,l1);
% C = subs(C,L2,l2);
% C = subs(C,L3,l3);
% C = subs(C,L4,l4);
% 
% C = subs(C,q1,q10);
% C = subs(C,q2,q20);
% C = subs(C,q3,q30);
% C = subs(C,q4,q40);
% 
% C = subs(C,diff(q1(t),t),w1);
% C = subs(C,diff(q2(t),t),w2);
% C = subs(C,diff(q3(t),t),w3);
% C = subs(C,diff(q4(t),t),w4);



tau = M*u+N;

== matlab function Leg/Control signal ==
  data: q_d input; dq_d input; u output; ddq_d input; q_a input; dq_a input
function u = fcn(q_d,dq_d,ddq_d, q_a,dq_a)
Kv=10;
Kp=15;
u = ddq_d + Kv*(dq_d-dq_a) + Kp*(q_d-q_a);
